simulink model "exerciseEx"  (R2022a)
settings: Solver=VariableStepAuto  StartTime=0.0  StopTime=10.0  RelTol=1e-3
libraries: cstblocks x2
settings Model: Creator=apple  LastModifiedBy=apple

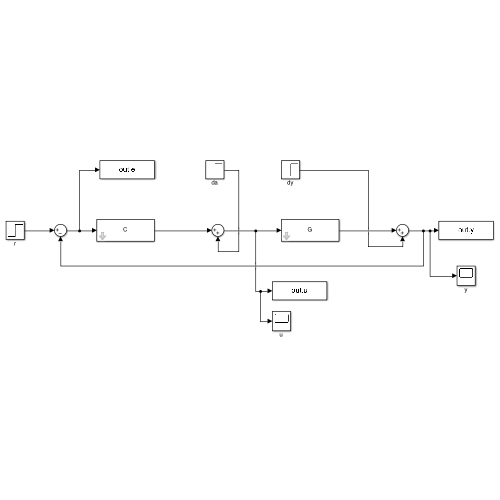
[thumbnail: Simulink's stored preview of the top-level diagram]
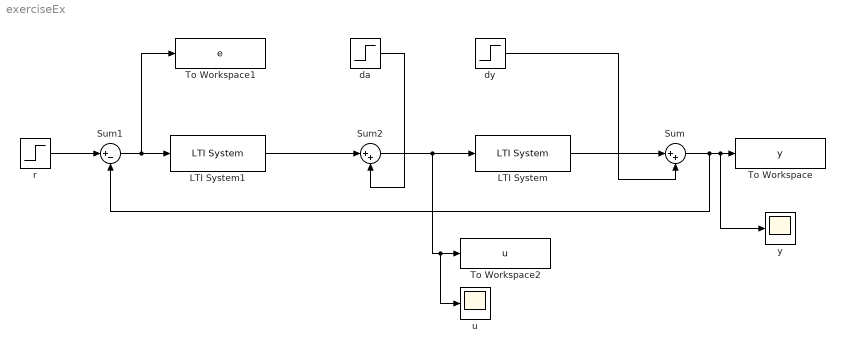
== system exerciseEx ==
  LTI System : cstblocks/LTI System  sys=G  IC=[]
  LTI System1 : cstblocks/LTI System  sys=C  IC=[]
  Sum : Sum  Inputs=|++
  Sum1 : Sum  Inputs=|+-
  Sum2 : Sum  Inputs=|++
  To Workspace : ToWorkspace  VariableName=y  SaveFormat=Timeseries  SampleTime=-1
  To Workspace1 : ToWorkspace  VariableName=e  SaveFormat=Timeseries  SampleTime=-1
  To Workspace2 : ToWorkspace  VariableName=u  SaveFormat=Timeseries  SampleTime=-1
  da : Step  Time=0  After=0  SampleTime=0
  dy : Step  Time=0  After=0  SampleTime=0
  r : Step  Time=0  SampleTime=0
  u : Scope
  y : Scope
  wires:
  r/1 -> Sum1/1
  Sum1/1 -> To Workspace1/1, LTI System1/1
  LTI System1/1 -> Sum2/1
  da/1 -> Sum2/2
  Sum2/1 -> u/1, To Workspace2/1, LTI System/1
  LTI System/1 -> Sum/1
  dy/1 -> Sum/2
  Sum/1 -> Sum1/2, y/1, To Workspace/1
